simulink model "FTTest05"  (R2013a)
settings: Solver=FixedStepDiscrete  StartTime=0.0  StopTime=inf  FixedStep=0.001  RelTol=1e-3
values from neighbouring files (symbols this model uses):
  s = double(D)    [parseFTCalibration.m]
undefined symbols (not defined in the file or in its folder): m_XR17D15x, MODBUS_TIMEOUT, standard, STREAMING_TIMEOUT
libraries: speedgoatlib x26, xpcseriallib x13, simulink x3, xpclib x1
settings Model: BufferReuse=off  Creator=bgbuss  LastModifiedBy=bgbuss
settings DataIOCC: LimitDataPoints=off
settings OptimizationCC: BlockReduction=off  OptimizeBlockIOStorage=off  BufferReuse=off  ExpressionFolding=off  LocalBlockOutputs=off
settings DebuggingCC: UnderspecifiedInitializationDetection=Simplified
settings HardwareCC: ProdIntDivRoundTo=Zero  ProdEndianess=LittleEndian  ProdHWDeviceType=Generic->32-bit x86 compatible
settings RTWCC: SystemTargetFile=xpctarget.tlc  TemplateMakefile=xpc_default_tmf  Description=xPC Target  ProcessScript=xpctarget_make_rtw_hook  RTWCompilerOptimization=On
settings CodeAppCC: MATLABSourceComments=on
settings xpcTargetCC: TargetFcnLib=ansi_tfl_table_tmw.mat  CodeReplacementLibrary=XPC_BLAS  ParMdlRefBuildCompliant=on  ConcurrentExecutionCompliant=on  CombineSignalStateStructs=off  MATLABClassNameForMDSCustomization=xpcAperiodicCustomization  GRTInterface=on  GenerateAllocFcn=off  RL32LogBufSizeModifier=100000000  xPCTaskExecutionProfile=off  xPCRL32EventNumber=5000  xPCisModelTimeout=off  xPCModelTimeoutSecs=20  xPCLoadParamSetFile=off  xPCConcurrentTasks=off  xPCEnableSFAnimation=off

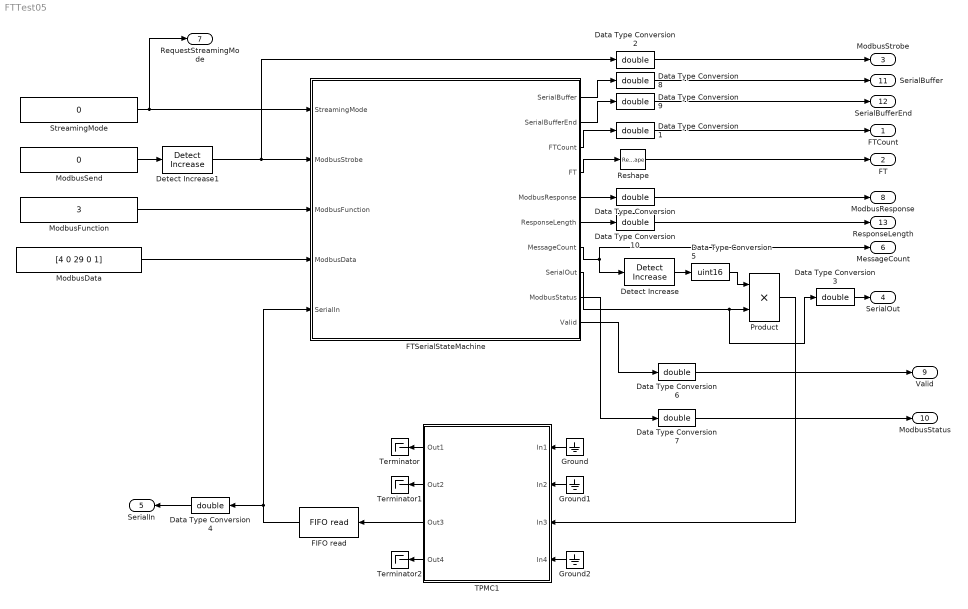
== system FTTest05 ==
  Data Type Conversion{,1..4,6..10} (10 alike) : DataTypeConversion  OutDataTypeStr=double
  Data Type Conversion5 : DataTypeConversion  OutDataTypeStr=uint16
  Detect Increase : simulink/Logic and Bit Operations/Detect Increase  vinit=0.0  InputProcessing=Inherited  OutDataTypeStr=uint8
  Detect Increase1 : simulink/Logic and Bit Operations/Detect Increase  vinit=0.0  InputProcessing=Inherited  OutDataTypeStr=uint8
  "FIFO read " : xpcseriallib/FIFO read   maxsize=255  minsize=1  usedelimiter=off  delimiter=13  outputtype=count+16 bit uint  enable=off  enableout=off  sampletime=0.001
  FTSerialStateMachine : Stateflow chart  TreatAsAtomicUnit=on
  Ground : Ground
  Ground1 : Ground
  Ground2 : Ground
  ModbusData : Constant  Value=[4 0 29 0 1]  OutDataTypeStr=uint16
  ModbusFunction : Constant  Value=3  OutDataTypeStr=uint16
  ModbusSend : Constant  Value=0  OutDataTypeStr=uint16
  Product : Product  OutDataTypeStr=uint16
  Reshape : Reshape
  StreamingMode : Constant  Value=0  OutDataTypeStr=double
  TPMC1 : Subsystem  AncestorBlock=speedgoatlib/IO503/TPMC466  InitFcn=m_XR17D15x(3);  mask(RS232 Send Receive){group=Basic Setup, port=3, irqnum=5, slot=[4 4], transceiver1=RS485 half-duplex, standard1=on, baud1=115200, bauddivisor1=1, sampling1=16x (standard), prescale1=off, parity1=None, ndata1=8, nstop1=1, rlevel1=1, hwmode1=none, swmode1=none, xonchar1=17, xoffchar1=19, rs485auto1=off, rs485delay1=0, xmtfifosize1=1024, xmtdatatype1=8 bit uint null terminated, rcvfifosize1=1024, transceiver2=RS232 (max 921.6kb/s), standard2=on, baud2=115200, bauddivisor2=1, sampling2=16x (standard), prescale2=off, parity2=None, ndata2=8, nstop2=1, rlevel2=1, hwmode2=none, swmode2=none, xonchar2=17, xoffchar2=19, rs485auto2=off, rs485delay2=0, xmtfifosize2=1024, xmtdatatype2=8 bit uint null terminated, rcvfifosize2=1024, transceiver3=RS485 half-duplex, standard3=on, baud3=1382400, bauddivisor3=1, sampling3=16x (standard), prescale3=off, parity3=Even, ndata3=8, nstop3=1, rlevel3=1, hwmode3=none, swmode3=none, xonchar3=17, xoffchar3=19, rs485auto3=on, rs485delay3=2, xmtfifosize3=128, xmtdatatype3=count+16 bit uint, rcvfifosize3=1024, transceiver4=RS232 (max 921.6kb/s), standard4=on, baud4=115200, bauddivisor4=1, sampling4=16x (standard), prescale4=off, parity4=None, ndata4=8, nstop4=1, rlevel4=half full (32), hwmode4=none, swmode4=none, xonchar4=17, xoffchar4=19, rs485auto4=off, rs485delay4=0, xmtfifosize4=1024, xmtdatatype4=8 bit uint null terminated, rcvfifosize4=1024}
      mask prompts: group "Parameter group:"; port "Port to modify:"; irqnum "IRQ number:"; slot "PCI slot (-1: autosearch):"; transceiver1 "Transceiver setup:"; standard1 "Use standard baud rates (16x, no prescaling)"; baud1 "Standard baud rate:"; bauddivisor1 "Baud rate divisor (non-standard baud rates):"; sampling1 "Sampling rate (non-standard baud rates):"; prescale1 "Prescale by 4 (non-standard baud rates)"; parity1 "Parity:"; ndata1 "Data bits:"; nstop1 "Stop bits:"; rlevel1 "Receive FIFO interrupt level:"; hwmode1 "Hardware handshake:"; swmode1 "Software handshake:"; xonchar1 "XON character:"; xoffchar1 "XOFF character:"; rs485auto1 "RS485 auto turnaround:"; rs485delay1 "RS485 turnaround delay [0,15]"; xmtfifosize1 "Transmit software FIFO size:"; xmtdatatype1 "Transmit FIFO data type:"; rcvfifosize1 "Receive software FIFO size:"; transceiver2 "Transceiver setup:"; standard2 "Use standard baud rates (16x, no prescaling)"; baud2 "Standard baud rate:"; bauddivisor2 "Baud rate divisor (non-standard baud rates):"; sampling2 "Sampling rate (non-standard baud rates):"; prescale2 "Prescale by 4 (non-standard baud rates)"; parity2 "Parity:"; ndata2 "Data bits:"; nstop2 "Stop bits:"; rlevel2 "Receive FIFO interrupt level:"; hwmode2 "Hardware handshake:"; swmode2 "Software handshake:"; xonchar2 "XON character:"; xoffchar2 "XOFF character:"; rs485auto2 "RS485 auto turnaround:"; rs485delay2 "RS485 turnaround delay [0,15]"; xmtfifosize2 "Transmit software FIFO size:"; xmtdatatype2 "Transmit FIFO data type:"; rcvfifosize2 "Receive software FIFO size:"; transceiver3 "Transceiver setup:"; standard3 "Use standard baud rates (16x, no prescaling)"; baud3 "Standard baud rate:"; bauddivisor3 "Baud rate divisor (non-standard baud rates):"; sampling3 "Sampling rate (non-standard baud rates):"; prescale3 "Prescale by 4 (non-standard baud rates)"; parity3 "Parity:"; ndata3 "Data bits:"; nstop3 "Stop bits:"; rlevel3 "Receive FIFO interrupt level:"; hwmode3 "Hardware handshake:"; swmode3 "Software handshake:"; xonchar3 "XON character:"; xoffchar3 "XOFF character:"; rs485auto3 "RS485 auto turnaround:"; rs485delay3 "RS485 turnaround delay [0,15]"; xmtfifosize3 "Transmit software FIFO size:"; xmtdatatype3 "Transmit FIFO data type:"; rcvfifosize3 "Receive software FIFO size:"; transceiver4 "Transceiver setup:"; standard4 "Use standard baud rates (16x, no prescaling)"; baud4 "Standard baud rate:"; bauddivisor4 "Baud rate divisor (non-standard baud rates):"; sampling4 "Sampling rate (non-standard baud rates):"; prescale4 "Prescale by 4 (non-standard baud rates)"; parity4 "Parity:"; ndata4 "Data bits:"; nstop4 "Stop bits:"; rlevel4 "Receive FIFO interrupt level:"; hwmode4 "Hardware handshake:"; swmode4 "Software handshake:"; xonchar4 "XON character:"; xoffchar4 "XOFF character:"; rs485auto4 "RS485 auto turnaround:"; rs485delay4 "RS485 turnaround delay [0,15]"; xmtfifosize4 "Transmit software FIFO size:"; xmtdatatype4 "Transmit FIFO data type:"; rcvfifosize4 "Receive software FIFO size:"
      mask help:
      | PMC521
      | Acromag
      | EIA/TIA-422B Send Receive Subsystem
      mask init:
      | brdslot = slot;
      | m_tews_XR17D15x(1, 4);
      mask Help: helpview(fullfile(docroot, 'mapfiles', 'xpc.map'), 'Commtech_Subsystem')
      mask TypeOptions group: Board Setup | Basic Setup | FIFO Setup
      mask Callback group: m_tews_XR17D15x(2, 4);
      mask TypeOptions port: 1 | 2 | 3 | 4
      mask Callback port: m_tews_XR17D15x(2, 4);
      mask TypeOptions transceiver1: RS232 (max 921.6kb/s) | RS422 | RS422 multidrop | RS485 full-duplex | RS485 half-duplex
      mask TypeOptions baud1: 2764800 | 1382400 | 921600 | 460800 | 230400 | 115200 | 57600 | 38400 | 19200 | 9600 | 4800 | 2400 | 1200 | 600 | 400
      mask TypeOptions sampling1: 8x | 16x (standard)
      mask TypeOptions parity1: None | Even | Odd | Mark | Space
      mask TypeOptions ndata1: 5 | 6 | 7 | 8
      mask TypeOptions nstop1: 1 | 2
      mask TypeOptions rlevel1: 1 | quarter full (16) | half full (32) | almost full (56)
      mask TypeOptions hwmode1: RTS/CTS | none
      mask TypeOptions swmode1: XON/XOFF | none
      mask TypeOptions xmtdatatype1: count+32 bit int | count+32 bit uint | count+16 bit int | count+16 bit uint | 8 bit int null terminated | 8 bit uint null terminated
      mask TypeOptions transceiver2: RS232 (max 921.6kb/s) | RS422 | RS422 multidrop | RS485 full-duplex | RS485 half-duplex
      mask TypeOptions baud2: 2764800 | 1382400 | 921600 | 460800 | 230400 | 115200 | 57600 | 38400 | 19200 | 9600 | 4800 | 2400 | 1200 | 600 | 400
      mask TypeOptions sampling2: 8x | 16x (standard)
      mask TypeOptions parity2: None | Even | Odd | Mark | Space
      mask TypeOptions ndata2: 5 | 6 | 7 | 8
      mask TypeOptions nstop2: 1 | 2
      mask TypeOptions rlevel2: 1 | quarter full (16) | half full (32) | almost full (56)
      mask TypeOptions hwmode2: RTS/CTS | none
      mask TypeOptions swmode2: XON/XOFF | none
      mask TypeOptions xmtdatatype2: count+32 bit int | count+32 bit uint | count+16 bit int | count+16 bit uint | 8 bit int null terminated | 8 bit uint null terminated
      mask TypeOptions transceiver3: RS232 (max 921.6kb/s) | RS422 | RS422 multidrop | RS485 full-duplex | RS485 half-duplex
      mask TypeOptions baud3: 2764800 | 1382400 | 921600 | 460800 | 230400 | 115200 | 57600 | 38400 | 19200 | 9600 | 4800 | 2400 | 1200 | 600 | 400
      mask TypeOptions sampling3: 8x | 16x (standard)
      mask TypeOptions parity3: None | Even | Odd | Mark | Space
      mask TypeOptions ndata3: 5 | 6 | 7 | 8
      mask TypeOptions nstop3: 1 | 2
      mask TypeOptions rlevel3: 1 | quarter full (16) | half full (32) | almost full (56)
      mask TypeOptions hwmode3: RTS/CTS | none
      mask TypeOptions swmode3: XON/XOFF | none
      mask TypeOptions xmtdatatype3: count+32 bit int | count+32 bit uint | count+16 bit int | count+16 bit uint | 8 bit int null terminated | 8 bit uint null terminated
      mask TypeOptions transceiver4: RS232 (max 921.6kb/s) | RS422 | RS422 multidrop | RS485 full-duplex | RS485 half-duplex
      mask TypeOptions baud4: 2764800 | 1382400 | 921600 | 460800 | 230400 | 115200 | 57600 | 38400 | 19200 | 9600 | 4800 | 2400 | 1200 | 600 | 400
      mask TypeOptions sampling4: 8x | 16x (standard)
      mask TypeOptions parity4: None | Even | Odd | Mark | Space
      mask TypeOptions ndata4: 5 | 6 | 7 | 8
      mask TypeOptions nstop4: 1 | 2
      mask TypeOptions rlevel4: 1 | quarter full (16) | half full (32) | almost full (56)
      mask TypeOptions hwmode4: RTS/CTS | none
      mask TypeOptions swmode4: XON/XOFF | none
      mask TypeOptions xmtdatatype4: count+32 bit int | count+32 bit uint | count+16 bit int | count+16 bit uint | 8 bit int null terminated | 8 bit uint null terminated
      mask Display:
      | disp('TEWS\nTPMC466\nRS232/422/485\nSend\nReceive');
      | port_label( 'input', 1, 'XMT1' );
      | port_label( 'input', 2, 'XMT2' );
      | port_label( 'input', 3, 'XMT3' );
      | port_label( 'input', 4, 'XMT4' );
      | 
      | port_label( 'output', 1, 'FIFO1' );
      | port_label( 'output', 2, 'FIFO2' );
      | port_label( 'output', 3, 'FIFO3' );
      | port_label( 'output', 4, 'FIFO4' );
  Terminator : Terminator
  Terminator1 : Terminator
  Terminator2 : Terminator
  FTCount : Outport
  FT : Outport  Port=2
  ModbusStrobe : Outport  Port=3
  SerialOut : Outport  Port=4
  SerialIn : Outport  Port=5
  MessageCount : Outport  Port=6
  RequestStreamingMode : Outport  Port=7
  ModbusResponse : Outport  Port=8
  Valid : Outport  Port=9
  ModbusStatus : Outport  Port=10
  SerialBuffer : Outport  Port=11
  SerialBufferEnd : Outport  Port=12
  ResponseLength : Outport  Port=13
  wires:
  FTSerialStateMachine/4(FT) -> Reshape/1
  Reshape/1 -> FT/1
  FTSerialStateMachine/3(FTCount) -> Data Type Conversion1/1
  TPMC1/3(Out3) -> "FIFO read "/1
  Product/1 -> TPMC1/3(In3)
  ModbusSend/1 -> Detect Increase1/1
  Detect Increase1/1 -> Data Type Conversion2/1, FTSerialStateMachine/2(ModbusStrobe)
  ModbusFunction/1 -> FTSerialStateMachine/3(ModbusFunction)
  ModbusData/1 -> FTSerialStateMachine/4(ModbusData)
  FTSerialStateMachine/5(ModbusResponse) -> Data Type Conversion/1
  TPMC1/1(Out1) -> Terminator/1
  TPMC1/2(Out2) -> Terminator1/1
  TPMC1/4(Out4) -> Terminator2/1
  Ground/1 -> TPMC1/1(In1)
  Ground2/1 -> TPMC1/4(In4)
  Ground1/1 -> TPMC1/2(In2)
  Data Type Conversion/1 -> ModbusResponse/1
  Data Type Conversion1/1 -> FTCount/1
  Data Type Conversion2/1 -> ModbusStrobe/1
  Data Type Conversion3/1 -> SerialOut/1
  "FIFO read "/1 -> Data Type Conversion4/1, FTSerialStateMachine/5(SerialIn)
  Data Type Conversion4/1 -> SerialIn/1
  FTSerialStateMachine/8(SerialOut) -> Data Type Conversion3/1, Product/2
  FTSerialStateMachine/7(MessageCount) -> MessageCount/1, Detect Increase/1
  Detect Increase/1 -> Data Type Conversion5/1
  Data Type Conversion5/1 -> Product/1
  StreamingMode/1 -> RequestStreamingMode/1, FTSerialStateMachine/1(StreamingMode)
  Data Type Conversion6/1 -> Valid/1
  FTSerialStateMachine/10(Valid) -> Data Type Conversion6/1
  Data Type Conversion7/1 -> ModbusStatus/1
  FTSerialStateMachine/9(ModbusStatus) -> Data Type Conversion7/1
  Data Type Conversion8/1 -> SerialBuffer/1
  FTSerialStateMachine/1(SerialBuffer) -> Data Type Conversion8/1
  Data Type Conversion9/1 -> SerialBufferEnd/1
  FTSerialStateMachine/2(SerialBufferEnd) -> Data Type Conversion9/1
  Data Type Conversion10/1 -> ResponseLength/1
  FTSerialStateMachine/6(ResponseLength) -> Data Type Conversion10/1

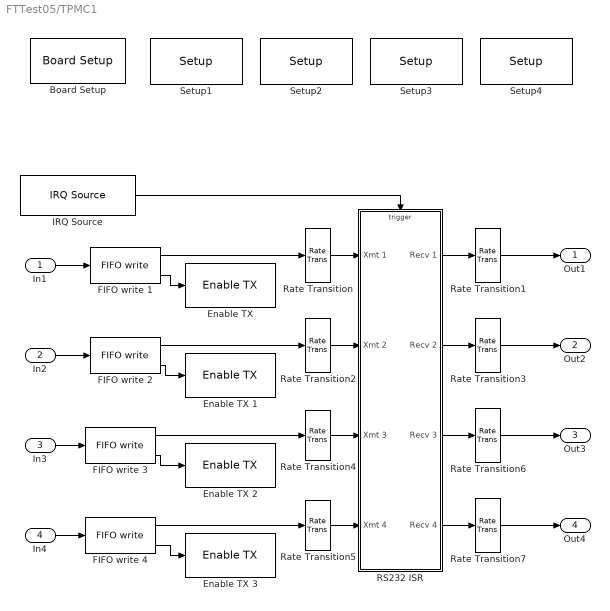
== system FTTest05/TPMC1 ==
  In1 : Inport
  In2 : Inport  Port=2
  In3 : Inport  Port=3
  In4 : Inport  Port=4
  Board Setup : speedgoatlib/IO503/TEWS TPMC466 Internal blocks/Board Setup  irqnum=5  slot=brdslot
  "Enable TX " : speedgoatlib/IO503/TEWS TPMC466 Internal blocks/Enable TX   port=1  slot=brdslot
  Enable TX 1 : speedgoatlib/IO503/TEWS TPMC466 Internal blocks/Enable TX   port=2  slot=brdslot
  Enable TX 2 : speedgoatlib/IO503/TEWS TPMC466 Internal blocks/Enable TX   port=3  slot=brdslot
  Enable TX 3 : speedgoatlib/IO503/TEWS TPMC466 Internal blocks/Enable TX   port=4  slot=brdslot
  FIFO write 1 : xpcseriallib/FIFO write   size=1024  inputtype=8 bit uint null terminated  present=on  sampletime=-1  id=XMT channel 1, IRQ 5
  FIFO write 2 : xpcseriallib/FIFO write   size=1024  inputtype=8 bit uint null terminated  present=on  sampletime=-1  id=XMT channel 2, IRQ 5
  FIFO write 3 : xpcseriallib/FIFO write   size=128  inputtype=count+16 bit uint  present=on  sampletime=-1  id=XMT channel 3, IRQ 5
  FIFO write 4 : xpcseriallib/FIFO write   size=1024  inputtype=8 bit uint null terminated  present=on  sampletime=-1  id=XMT channel 4, IRQ 5
  IRQ Source : xpclib/Asynchronous Event/IRQ Source  irqNo=5  preempt=off  b_type=None/Other  slot=brdslot
  RS232 ISR : Subsystem  TreatAsAtomicUnit=on  mask(RS232 ISR){slot=brdslot}
      mask help:
      | PMC521
      | Acromag
      | Interrupt Service Routine
      mask init:
      | subslot = slot;
      mask Display:
      | disp('PMC521\nAcromag\nISR');
      | port_label('input', 1, 'XMT1');
      | port_label('input', 2, 'XMT2');
      | port_label('input', 3, 'XMT3');
      | port_label('input', 4, 'XMT4');
      | port_label('input', 5, 'XMT5');
      | port_label('input', 6, 'XMT6');
      | port_label('input', 7, 'XMT7');
      | port_label('input', 8, 'XMT8');
      | port_label('output', 1, 'RCV1');
      | port_label('output', 2, 'RCV2');
      | port_label('output', 3, 'RCV3');
      | port_label('output', 4, 'RCV4');
      | port_label('output', 5, 'RCV5');
      | port_label('output', 6, 'RCV6');
      | port_label('output', 7, 'RCV7');
      | port_label('output', 8, 'RCV8');
  Rate Transition{,2,4..5} (4 alike) : RateTransition  Integrity=off  Deterministic=off
  Rate Transition{1,3,6..7} (4 alike) : RateTransition  Integrity=off  Deterministic=off  OutPortSampleTime=0
  Setup1 : speedgoatlib/IO503/TEWS TPMC466 Internal blocks/Setup   port=1  transceiver=RS485 half-duplex  standard=on  baudrate=115200  bauddivisor=1  mode8x=16x (standard)  prescale=off  width=8  nstop=1  parity=None  rlevel=1  ctsmode=none  xonoff=none  xon=17  xoff=19  rs485mode=off  rs485delay=0  slot=brdslot
  Setup2 : speedgoatlib/IO503/TEWS TPMC466 Internal blocks/Setup   port=2  transceiver=RS232 (max 921.6kb/s)  standard=on  baudrate=115200  bauddivisor=1  mode8x=16x (standard)  prescale=off  width=8  nstop=1  parity=None  rlevel=1  ctsmode=none  xonoff=none  xon=17  xoff=19  rs485mode=off  rs485delay=0  slot=brdslot
  Setup3 : speedgoatlib/IO503/TEWS TPMC466 Internal blocks/Setup   port=3  transceiver=RS485 half-duplex  standard=on  baudrate=1382400  bauddivisor=1  mode8x=16x (standard)  prescale=off  width=8  nstop=1  parity=Even  rlevel=1  ctsmode=none  xonoff=none  xon=17  xoff=19  rs485mode=on  rs485delay=2  slot=brdslot
  Setup4 : speedgoatlib/IO503/TEWS TPMC466 Internal blocks/Setup   port=4  transceiver=RS232 (max 921.6kb/s)  standard=on  baudrate=115200  bauddivisor=1  mode8x=16x (standard)  prescale=off  width=8  nstop=1  parity=None  rlevel=half full (32)  ctsmode=none  xonoff=none  xon=17  xoff=19  rs485mode=off  rs485delay=0  slot=brdslot
  Out1 : Outport
  Out2 : Outport  Port=2
  Out3 : Outport  Port=3
  Out4 : Outport  Port=4
  wires:
  RS232 ISR/4(Recv 4) -> Rate Transition7/1
  RS232 ISR/3(Recv 3) -> Rate Transition6/1
  Rate Transition7/1 -> Out4/1
  Rate Transition6/1 -> Out3/1
  Rate Transition5/1 -> RS232 ISR/4(Xmt 4)
  Rate Transition4/1 -> RS232 ISR/3(Xmt 3)
  FIFO write 4/1 -> Rate Transition5/1
  In4/1 -> FIFO write 4/1
  FIFO write 4/2 -> Enable TX 3/1
  FIFO write 3/1 -> Rate Transition4/1
  In3/1 -> FIFO write 3/1
  FIFO write 3/2 -> Enable TX 2/1
  Rate Transition1/1 -> Out1/1
  Rate Transition3/1 -> Out2/1
  Rate Transition/1 -> RS232 ISR/1(Xmt 1)
  Rate Transition2/1 -> RS232 ISR/2(Xmt 2)
  FIFO write 1/2 -> "Enable TX "/1
  IRQ Source/1 -> RS232 ISR/Trigger
  RS232 ISR/1(Recv 1) -> Rate Transition1/1
  RS232 ISR/2(Recv 2) -> Rate Transition3/1
  FIFO write 1/1 -> Rate Transition/1
  In1/1 -> FIFO write 1/1
  FIFO write 2/1 -> Rate Transition2/1
  In2/1 -> FIFO write 2/1
  FIFO write 2/2 -> Enable TX 1/1

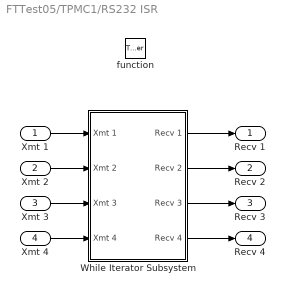
== system FTTest05/TPMC1/RS232 ISR ==
  Xmt 1 : Inport
  Xmt 2 : Inport  Port=2
  Xmt 3 : Inport  Port=3
  Xmt 4 : Inport  Port=4
  function : TriggerPort  TriggerType=function-call
  While Iterator Subsystem : Subsystem  TreatAsAtomicUnit=on
  Recv 1 : Outport  SourceOfInitialOutputValue=Input signal
  Recv 2 : Outport  Port=2  SourceOfInitialOutputValue=Input signal
  Recv 3 : Outport  Port=3  SourceOfInitialOutputValue=Input signal
  Recv 4 : Outport  Port=4  SourceOfInitialOutputValue=Input signal
  wires:
  While Iterator Subsystem/4(Recv 4) -> Recv 4/1
  While Iterator Subsystem/3(Recv 3) -> Recv 3/1
  Xmt 4/1 -> While Iterator Subsystem/4(Xmt 4)
  Xmt 3/1 -> While Iterator Subsystem/3(Xmt 3)
  While Iterator Subsystem/2(Recv 2) -> Recv 2/1
  While Iterator Subsystem/1(Recv 1) -> Recv 1/1
  Xmt 2/1 -> While Iterator Subsystem/2(Xmt 2)
  Xmt 1/1 -> While Iterator Subsystem/1(Xmt 1)

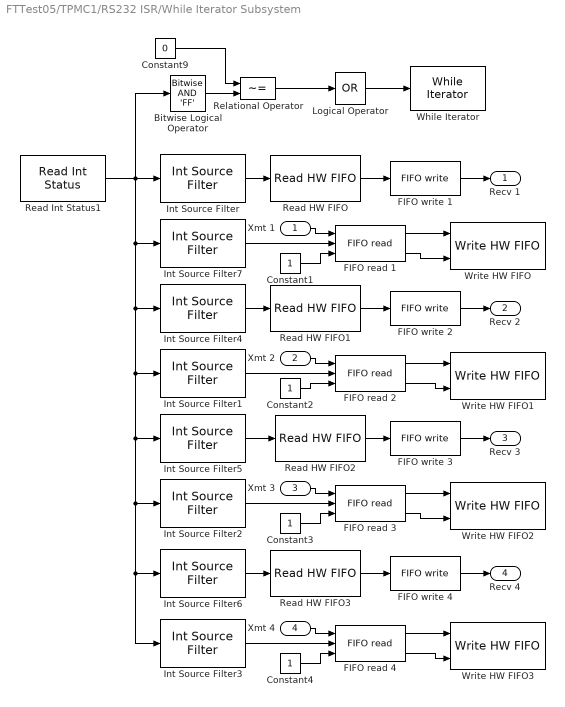
== system FTTest05/TPMC1/RS232 ISR/While Iterator Subsystem ==
  Xmt 1 : Inport
  Xmt 2 : Inport  Port=2
  Xmt 3 : Inport  Port=3
  Xmt 4 : Inport  Port=4
  Bitwise Logical Operator : simulink/Logic and Bit Operations/Bitwise Operator  logicop=AND  UseBitMask=on  BitMask='FF'  BitMaskRealWorld=Stored Integer
  Constant{1..4} (4 alike) : Constant  OutDataTypeStr=uint32
  Constant9 : Constant  Value=0  OutDataTypeStr=uint32
  FIFO read {1..4} (4 alike) : xpcseriallib/FIFO read   maxsize=60  minsize=1  usedelimiter=off  delimiter=13  outputtype=count+32 bit uint  enable=on  enableout=on  sampletime=-1
  FIFO write 1 : xpcseriallib/FIFO write   size=1024  inputtype=count+32 bit uint  present=off  sampletime=-1  id=RCV channel 1, IRQ 5
  FIFO write 2 : xpcseriallib/FIFO write   size=1024  inputtype=count+32 bit uint  present=off  sampletime=-1  id=RCV channel 2, IRQ 5
  FIFO write 3 : xpcseriallib/FIFO write   size=1024  inputtype=count+32 bit uint  present=off  sampletime=-1  id=RCV channel 3, IRQ 5
  FIFO write 4 : xpcseriallib/FIFO write   size=1024  inputtype=count+32 bit uint  present=off  sampletime=-1  id=RCV channel 4, IRQ 5
  Int Source Filter : speedgoatlib/IO503/TEWS TPMC466 Internal blocks/Int Source Filter  port=1  value=Receive data
  Int Source Filter1 : speedgoatlib/IO503/TEWS TPMC466 Internal blocks/Int Source Filter  port=2  value=Transmitter empty
  Int Source Filter2 : speedgoatlib/IO503/TEWS TPMC466 Internal blocks/Int Source Filter  port=3  value=Transmitter empty
  Int Source Filter3 : speedgoatlib/IO503/TEWS TPMC466 Internal blocks/Int Source Filter  port=4  value=Transmitter empty
  Int Source Filter4 : speedgoatlib/IO503/TEWS TPMC466 Internal blocks/Int Source Filter  port=2  value=Receive data
  Int Source Filter5 : speedgoatlib/IO503/TEWS TPMC466 Internal blocks/Int Source Filter  port=3  value=Receive data
  Int Source Filter6 : speedgoatlib/IO503/TEWS TPMC466 Internal blocks/Int Source Filter  port=4  value=Receive data
  Int Source Filter7 : speedgoatlib/IO503/TEWS TPMC466 Internal blocks/Int Source Filter  port=1  value=Transmitter empty
  Logical Operator : Logic  Operator=OR  Inputs=1  AllPortsSameDT=off
  Read HW FIFO : speedgoatlib/IO503/TEWS TPMC466 Internal blocks/Read HW FIFO  port=1  flush=on  slot=subslot
  Read HW FIFO1 : speedgoatlib/IO503/TEWS TPMC466 Internal blocks/Read HW FIFO  port=2  flush=on  slot=subslot
  Read HW FIFO2 : speedgoatlib/IO503/TEWS TPMC466 Internal blocks/Read HW FIFO  port=3  flush=on  slot=subslot
  Read HW FIFO3 : speedgoatlib/IO503/TEWS TPMC466 Internal blocks/Read HW FIFO  port=4  flush=on  slot=subslot
  Read Int Status1 : speedgoatlib/IO503/TEWS TPMC466 Internal blocks/Read Int Status  slot=subslot
  Relational Operator : RelationalOperator  Operator=~=
  While Iterator : WhileIterator  MaxIters=65  WhileBlockType=do-while
  Write HW FIFO : speedgoatlib/IO503/TEWS TPMC466 Internal blocks/Write HW FIFO  port=1  slot=subslot
  Write HW FIFO1 : speedgoatlib/IO503/TEWS TPMC466 Internal blocks/Write HW FIFO  port=2  slot=subslot
  Write HW FIFO2 : speedgoatlib/IO503/TEWS TPMC466 Internal blocks/Write HW FIFO  port=3  slot=subslot
  Write HW FIFO3 : speedgoatlib/IO503/TEWS TPMC466 Internal blocks/Write HW FIFO  port=4  slot=subslot
  Recv 1 : Outport  SourceOfInitialOutputValue=Input signal
  Recv 2 : Outport  Port=2  SourceOfInitialOutputValue=Input signal
  Recv 3 : Outport  Port=3  SourceOfInitialOutputValue=Input signal
  Recv 4 : Outport  Port=4  SourceOfInitialOutputValue=Input signal
  wires:
  Read HW FIFO3/1 -> FIFO write 4/1
  FIFO write 4/1 -> Recv 4/1
  Read HW FIFO2/1 -> FIFO write 3/1
  FIFO write 3/1 -> Recv 3/1
  Int Source Filter6/1 -> Read HW FIFO3/1
  Int Source Filter5/1 -> Read HW FIFO2/1
  Constant3/1 -> FIFO read 3/3
  FIFO read 3/2 -> Write HW FIFO2/2
  FIFO read 3/1 -> Write HW FIFO2/1
  Xmt 3/1 -> FIFO read 3/1
  Int Source Filter2/1 -> FIFO read 3/2
  Constant2/1 -> FIFO read 2/3
  Constant1/1 -> FIFO read 1/3
  FIFO read 2/2 -> Write HW FIFO1/2
  FIFO read 1/2 -> Write HW FIFO/2
  FIFO read 1/1 -> Write HW FIFO/1
  FIFO read 2/1 -> Write HW FIFO1/1
  Xmt 2/1 -> FIFO read 2/1
  Int Source Filter1/1 -> FIFO read 2/2
  Read HW FIFO1/1 -> FIFO write 2/1
  FIFO write 2/1 -> Recv 2/1
  Int Source Filter4/1 -> Read HW FIFO1/1
  Xmt 1/1 -> FIFO read 1/1
  Int Source Filter7/1 -> FIFO read 1/2
  Read HW FIFO/1 -> FIFO write 1/1
  FIFO write 1/1 -> Recv 1/1
  Int Source Filter/1 -> Read HW FIFO/1
  Read Int Status1/1 -> Bitwise Logical Operator/1, Int Source Filter6/1, Int Source Filter3/1, Int Source Filter2/1, Int Source Filter5/1, Int Source Filter1/1, Int Source Filter4/1, Int Source Filter7/1, Int Source Filter/1
  Constant9/1 -> Relational Operator/1
  Bitwise Logical Operator/1 -> Relational Operator/2
  Relational Operator/1 -> Logical Operator/1
  Logical Operator/1 -> While Iterator/1
  Constant4/1 -> FIFO read 4/3
  FIFO read 4/2 -> Write HW FIFO3/2
  FIFO read 4/1 -> Write HW FIFO3/1
  Xmt 4/1 -> FIFO read 4/1
  Int Source Filter3/1 -> FIFO read 4/2

== stateflow chart FTTest05/FTSerialStateMachine ==
  state StreamingMode
    en:
    clearFT();
    clearSerialOut();
    clearSerialBuffer();
    du:
    parseStreamingData();
  state ModbusMode
    en:
    clearFT();
    clearSerialOut();
    MessageCount = 0;
    state ModbusIdle
      entry:
      clearSerialBuffer();
    state ModbusSend
      entry:
      sendModbusCmd(ModbusFunction, ModbusData);
      exit:
      clearSerialOut();
    state ModbusReceive
      entry, during:
      readModbusResponse()
    state ModbusValidate
      entry:
      validateModbusResponse();
      exit:
      clearModbusResponse();
    (default) -> ModbusIdle
    (junction 37) -> ModbusIdle
    (junction 36) -> (junction 37)
    ModbusIdle -> ModbusSend [order 2] : [ModbusStrobe==1]
    ModbusSend -> ModbusReceive
    ModbusReceive -> (junction 36) [order 2] : [after(MODBUS_TIMEOUT, sec)]
    (junction 86) -> (junction 36)
    ModbusReceive -> ModbusValidate [order 1] : [ModbusStatus~=0]
    ModbusValidate -> (junction 86)
  state InitializeStreaming
    entry:
    clearSerialBuffer();
    sendStreamingCmd(1);
    exit:
    clearSerialOut();
  state CheckStreaming
    state WaitClear
      entry:
      clearSerialOut();
      clearSerialBuffer();
    state CheckSerialInput
    (default) -> WaitClear
    WaitClear -> CheckSerialInput
  state EndStreaming
    entry:
    clearSerialBuffer();
    sendStreamingCmd(0);
    exit:
    clearSerialOut();
  ModbusIdle -> InitializeStreaming [order 1] : [StreamingMode~=0]
  InitializeStreaming -> CheckStreaming
  (default) -> CheckStreaming
  CheckSerialInput -> ModbusMode [order 2] : [after(STREAMING_TIMEOUT, sec)]
  CheckSerialInput -> StreamingMode [order 1] : [SerialIn(1)>0]
  EndStreaming -> CheckStreaming
  StreamingMode -> EndStreaming : [StreamingMode==0]
  data: Function function_input; Data function_input; Select function_input; StreamingMode input; ModbusStrobe input; SerialBuffer output; SerialBufferEnd output; FTCount output; FT output size=[6 8]; ModbusFunction input; ModbusResponse output; ModbusData input; SerialIn input uint16; ResponseLength output; MessageCount output; SerialOut output; LastModbusFunction local; ModbusStatus output; MODBUS_TIMEOUT parameter; STREAMING_TIMEOUT parameter; Valid output
  function parseStreamingData:
    | function parseStreamingData %#codegen
    |     [FTCount, FT, SerialBuffer, SerialBufferEnd] = parseStreamingFTData(SerialIn, SerialBuffer, SerialBufferEnd);
    | end
  function clearSerialOut:
    | function clearSerialOut %#codegen
    |     SerialOut = zeros(256,1, 'uint16');
    | end
  function sendModbusCmd(Function, Data):
    | function sendModbusCmd(Function, Data) %#codegen
    |     
    |     % All ATI Digital F/T interface boards use Modbus address 10.
    |     % See ATI Digital F/T System Installation and Operation Manual
    |     % (Document #9620-05-Digital FT).
    |     ModbusAddress = uint16(10); 
    |     ModbusPacket = createModbusPacket(ModbusAddress, Function, Data(1+(1:Data(1))));
    |     
    |     L = length(ModbusPacket);
    |     SerialOut(1)     = uint16(L);
    |     SerialOut(2:L+1) = ModbusPacket;
    |     
    |     % Expected response length
    |     ResponseLength = getModbusResponseLength(ModbusFunction, ModbusData);
    |     
    |     % Increment message counter
    |     % This serves to indicate that a new message is to be sent to the
    |     % Modbus slave
    |     MessageCount = MessageCount + 1;
    |     
    |     % Capture function
    |     LastModbusFunction = ModbusFunction;
    | end
  function sendStreamingCmd(Select):
    | function sendStreamingCmd(Select) %#codegen
    |     
    |     Function = uint16(70);
    |     if (Select==1)
    |         Data = uint16([1; 85]);
    |     else
    |         Data = [uint16(15); 85*ones(15,1,'uint16')]; % JAMMING SEQUENCE
    |     end
    |     sendModbusCmd(Function, Data) %#codegen
    | end
  function clearFT:
    | function clearFT %#codegen
    |     FT = zeros(6,8);
    |     FTCount = 0;
    | end
  function readModbusResponse:
    | function readModbusResponse %#codegen
    |     [ModbusStatus, SerialBuffer, SerialBufferEnd] = bufferModbusData(LastModbusFunction, ResponseLength, SerialIn, SerialBuffer, SerialBufferEnd);
    | end
  function validateModbusResponse:
    | function validateModbusResponse %#codegen
    |     Valid = false;
    |     ModbusResponse = zeros(256,1,'uint16');
    |     
    |     if (SerialBuffer(2) == LastModbusFunction) && (SerialBufferEnd == 3 + ResponseLength) ...
    |             || (SerialBuffer(2) == ModbusFunction + 128) && (SerialBufferEnd == 5)
    |         
    |         Valid = checkModbusCRC(SerialBuffer(1:SerialBufferEnd));
    |         if Valid
    |             % Strip off the Modbus Address and CRC
    |             L = SerialBufferEnd-3;
    |             ModbusResponse(1) = uint16(L);
    |             ModbusResponse(1+(1:L)) = SerialBuffer(1+(1:L));
    |             %MessageCount = MessageCount + 1;
    |         end
    |     end
    | end
  function clearSerialBuffer:
    | function clearSerialBuffer %#codegen
    |     SerialBuffer = zeros(512,1,'uint16');
    |     SerialBufferEnd = uint16(0);
    | end
  function clearModbusResponse:
    | function clearModbusResponse %#codegen
    |     ModbusResponse(1) = uint16(0);
    | end
